simulink model "NL_Trajectory_Tracking_and_Posture_Regulation2_2024b"  (R2025b)
settings: Solver=FixedStepAuto  StartTime=0.0  StopTime=30  FixedStep=0.001  RelTol=1e-3
values from neighbouring files (symbols this model uses):
  b = 3    [NonLin_Traj_params.mat]    (also in compare_methods.m = 15; simulation.m = 500; tuning_simulation.m = 0.005)
  k1 = 0.5    [Posture_gains.mat]    (also in simulation.m = 1.5)
  k2 = 5    [Posture_gains.mat]    (also in simulation.m = 4)
  k3 = 2    [Posture_gains.mat]    (also in simulation.m = 1.5)
  last_t = size(xy, 1)-1    [simulation.m]
  theta0 = -pi/2    (= -1.57079632679)    [automated_tuning_simulation.m]    (also in regulation_tuning_simulation.m = 0.785398163397; simulation.m = 0.785398163397; tuning_simulation.m = 0.785398163397)
  x0 = S.traj.xy(1,1)    [automated_tuning_simulation.m]    (also in regulation_tuning_simulation.m = -0.8; simulation.m; tuning_simulation.m)
  x_box = 850    [parking_box.mat]    (also in regulation_tuning_simulation.m = 0; replay_q_timeseries_on_maze_pacman.m; replay_q_timeseries_on_maze_pacman_real.m; simulation.m)
  xi = 0.7    [Lin_Traj_params.mat]    (also in NonLin_Traj_params.mat = 0.706; automated_tuning_simulation.m = XI_test(j); compare_methods.m = 0.706; simulation.m)
  y0 = S.traj.xy(1,2)    [automated_tuning_simulation.m]    (also in regulation_tuning_simulation.m = 0.5; simulation.m; tuning_simulation.m)
  y_box = 880    [parking_box.mat]    (also in regulation_tuning_simulation.m = 0; replay_q_timeseries_on_maze_pacman.m; replay_q_timeseries_on_maze_pacman_real.m; simulation.m)
settings Model: Creator=david  LastModifiedBy=david
settings DataIOCC: ReturnWorkspaceOutputs=off

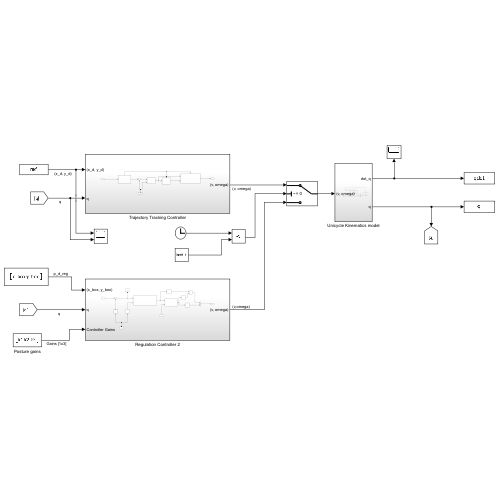
[thumbnail: Simulink's stored preview of the top-level diagram]
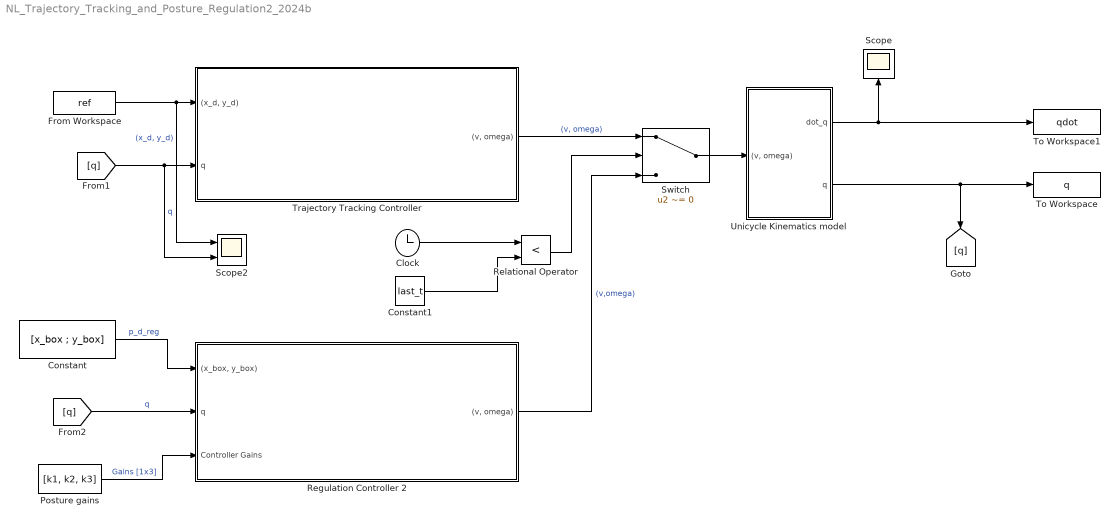
== system NL_Trajectory_Tracking_and_Posture_Regulation2_2024b ==
  Clock : Clock
  Constant : Constant  Value=[x_box ; y_box]
  Constant1 : Constant  Value=last_t
  From Workspace : FromWorkspace  VariableName=ref  OutDataTypeStr=double  SampleTime=-1
  Posture gains : Constant  Value=[k1, k2, k3]
  Regulation Controller 2 : Subsystem
  Relational Operator : RelationalOperator  Operator=<  OutDataTypeStr=boolean  RndMeth=Simplest  InputSameDT=off
  Scope : Scope
      settings: ActiveDisplayYMinimum=-1203.295  ActiveDisplayYMaximum=630.9359
  Scope2 : Scope  NumInputPorts=2
      settings: ActiveDisplayYMinimum=-704.7353  ActiveDisplayYMaximum=6091.8367  DataLoggingVariableName=ScopeData2
  Switch : Switch  Criteria=u2 ~= 0  Threshold=110  SaturateOnIntegerOverflow=off  InputSameDT=off
  To Workspace : ToWorkspace  VariableName=q  SaveFormat=Timeseries  SampleTime=-1
  To Workspace1 : ToWorkspace  VariableName=qdot  SaveFormat=Timeseries  SampleTime=-1
  Trajectory Tracking Controller : Subsystem
  Unicycle Kinematics model : Subsystem
  wires:
  Constant/1 -> Regulation Controller 2/1("(x_box, y_box)")  "p_d_reg"
  Unicycle Kinematics model/2(q) -> To Workspace/1, [q]
  From Workspace/1 -> Scope2/1, Trajectory Tracking Controller/1("(x_d, y_d)")  "(x_d, y_d)"
  Switch/1 -> Unicycle Kinematics model/1("(v, omega)")
  [q] -> Scope2/2, Trajectory Tracking Controller/2(q)  "q"
  Trajectory Tracking Controller/1("(v, omega)") -> Switch/1  "(v, omega)"
  Relational Operator/1 -> Switch/2
  Unicycle Kinematics model/1(dot_q) -> Scope/1, To Workspace1/1
  Regulation Controller 2/1("(v, omega)") -> Switch/3  "(v,omega)"
  Clock/1 -> Relational Operator/1
  Posture gains/1 -> Regulation Controller 2/3(Controller Gains)  "Gains [1x3]"
  [q] -> Regulation Controller 2/2(q)  "q"
  Constant1/1 -> Relational Operator/2

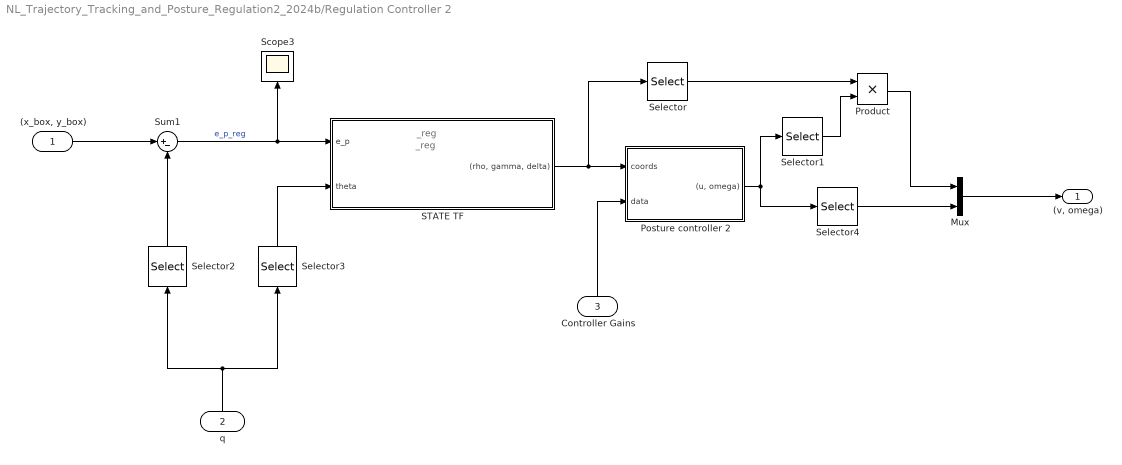
== system NL_Trajectory_Tracking_and_Posture_Regulation2_2024b/Regulation Controller 2 ==
  note: _reg
  note: _reg
  "(x_box, y_box)" : Inport
  q : Inport  Port=2
  Controller Gains : Inport  Port=3
  Mux : Mux  Inputs=2
  Posture controller 2 : Subsystem
  Product : Product
  "STATE TF " : Subsystem
  Scope3 : Scope
      settings: ActiveDisplayYMinimum=-1.51842483246E+7  ActiveDisplayYMaximum=1.6973761395E+6  DataLoggingVariableName=ScopeData3
  Selector : Selector  InputPortWidth=3  IndexOptions=Index vector (dialog)  Indices=[1]  OutputSizes=1
  Selector1 : Selector  InputPortWidth=2  IndexOptions=Index vector (dialog)  Indices=[1]  OutputSizes=1
  Selector2 : Selector  InputPortWidth=3  IndexOptions=Index vector (dialog)  Indices=[1 2]  OutputSizes=1
  Selector3 : Selector  InputPortWidth=3  IndexOptions=Index vector (dialog)  Indices=[3]  OutputSizes=1
  Selector4 : Selector  InputPortWidth=2  IndexOptions=Index vector (dialog)  Indices=[2]  OutputSizes=1
  Sum1 : Sum  Inputs=|+-
  "(v, omega)" : Outport
  wires:
  Selector2/1 -> Sum1/2
  Sum1/1 -> "STATE TF "/1(e_p), Scope3/1  "e_p_reg"
  Selector3/1 -> "STATE TF "/2(theta)
  "STATE TF "/1("(rho, gamma, delta)") -> Selector/1, Posture controller 2/1(coords)
  q/1 -> Selector3/1, Selector2/1
  Controller Gains/1 -> Posture controller 2/2(data)
  "(x_box, y_box)"/1 -> Sum1/1
  Selector/1 -> Product/1
  Selector1/1 -> Product/2
  Posture controller 2/1("(u, omega)") -> Selector4/1, Selector1/1
  Mux/1 -> "(v, omega)"/1
  Product/1 -> Mux/1
  Selector4/1 -> Mux/2

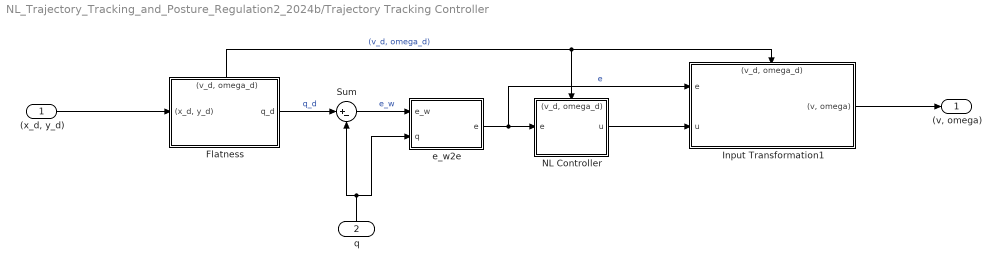
== system NL_Trajectory_Tracking_and_Posture_Regulation2_2024b/Trajectory Tracking Controller ==
  "(x_d, y_d)" : Inport
  q : Inport  Port=2
  Flatness : Subsystem
      settings: PortSchema="{\"entries\":[{\"content\":{\"sides\":[{\"content\":{\"connectorIds\":[\"In1\"]},\"type\":\"ConnectorPlacement.EquallySpacedRectSide\",\"uuid\":\"bc490c8e-5666-439b-9939-62bd84628b1f\"},{\"content\":{\"connectorIds\":[\"Out1\"],\"side\":\"RIGHT\"},\"type\":\"ConnectorPlacement.EquallySpacedRectSide\",\"uuid\":\"03a20fcc-2a82-4af2-a970-ff3426fda7d9\"},{\"content\":{\"connectorIds\":[\"Out2\"],\"side\":\"TOP\"},\"type\":\"ConnectorPlacement.EquallySpacedRectSide\",\"uuid\":\"09224fef-e39c-4959-bd2b-02867a510190\"}]},\"type\":\"ConnectorPlacement.EquallySpacedConnector\",\"uuid\":\"ad9510e9-14f7-413e-ab85-da35fb962608\"}],\"packageUris\":[\"http://schema.mathworks.com/mf0/Connector/R2020b\"],\"version\":\"1.0\"}"
  Input Transformation1 : Subsystem
      settings: PortSchema="{\"entries\":[{\"content\":{\"sides\":[{\"content\":{\"connectorIds\":[\"In1\",\"In2\"]},\"type\":\"ConnectorPlacement.EquallySpacedRectSide\",\"uuid\":\"4cbebdc1-8913-4bb0-9524-d854c819f784\"},{\"content\":{\"connectorIds\":[\"Out1\"],\"side\":\"RIGHT\"},\"type\":\"ConnectorPlacement.EquallySpacedRectSide\",\"uuid\":\"178a2b4a-0c33-47f3-8be3-bd76dfc47961\"},{\"content\":{\"connectorIds\":[\"In3\"],\"side\":\"TOP\"},\"type\":\"ConnectorPlacement.EquallySpacedRectSide\",\"uuid\":\"3e37ae07-0719-4d1d-ac53-f79374967c51\"}]},\"type\":\"ConnectorPlacement.EquallySpacedConnector\",\"uuid\":\"35111781-18f4-42cf-8750-882b65aa13c0\"}],\"packageUris\":[\"http://schema.mathworks.com/mf0/Connector/R2020b\"],\"version\":\"1.0\"}"
  NL Controller : Subsystem
      settings: PortSchema="{\"entries\":[{\"content\":{\"sides\":[{\"content\":{\"connectorIds\":[\"In1\"]},\"type\":\"ConnectorPlacement.EquallySpacedRectSide\",\"uuid\":\"111a75b0-1720-417b-bb3b-4eef3b94ce3e\"},{\"content\":{\"connectorIds\":[\"Out1\"],\"side\":\"RIGHT\"},\"type\":\"ConnectorPlacement.EquallySpacedRectSide\",\"uuid\":\"fd08faf2-16f9-4b1a-8555-2743d2eb322e\"},{\"content\":{\"connectorIds\":[\"In2\"],\"side\":\"TOP\"},\"type\":\"ConnectorPlacement.EquallySpacedRectSide\",\"uuid\":\"17cbf3ba-8c3f-4714-857c-1066f0d359bd\"}]},\"type\":\"ConnectorPlacement.EquallySpacedConnector\",\"uuid\":\"cf97b092-2f26-4cb4-9c58-7f62a3040eca\"}],\"packageUris\":[\"http://schema.mathworks.com/mf0/Connector/R2020b\"],\"version\":\"1.0\"}"
  Sum : Sum  Inputs=|+-
  e_w2e : MATLAB Function  TreatAsAtomicUnit=on
  "(v, omega)" : Outport
  wires:
  q/1 -> e_w2e/2(q), Sum/2
  NL Controller/1(u) -> Input Transformation1/2(u)
  e_w2e/1(e) -> NL Controller/1(e), Input Transformation1/1(e)  "e"
  Sum/1 -> e_w2e/1(e_w)  "e_w"
  Input Transformation1/1("(v, omega)") -> "(v, omega)"/1
  Flatness/2("(v_d, omega_d)") -> Input Transformation1/3("(v_d, omega_d)"), NL Controller/2("(v_d, omega_d)")  "(v_d, omega_d)"
  Flatness/1(q_d) -> Sum/1  "q_d"
  "(x_d, y_d)"/1 -> Flatness/1("(x_d, y_d)")

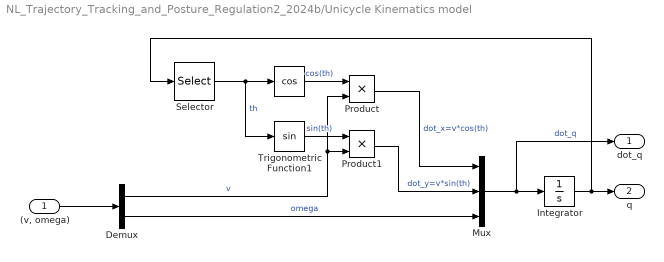
== system NL_Trajectory_Tracking_and_Posture_Regulation2_2024b/Unicycle Kinematics model ==
  "(v, omega)" : Inport
  " " : Trigonometry  Operator=cos
  Demux : Demux  Outputs=2
  Integrator : Integrator  InitialCondition=[x0; y0; theta0]
  Mux : Mux  Inputs=3
  Product : Product
  Product1 : Product
  Selector : Selector  InputPortWidth=3  IndexOptions=Index vector (dialog)  Indices=[3]  OutputSizes=1
  Trigonometric Function1 : Trigonometry
  dot_q : Outport
  q : Outport  Port=2
  wires:
  Integrator/1 -> Selector/1, q/1
  "(v, omega)"/1 -> Demux/1
  Mux/1 -> Integrator/1, dot_q/1  "dot_q"
  Demux/2 -> Mux/3  "omega"
  Selector/1 -> Trigonometric Function1/1, " "/1  "th"
  " "/1 -> Product/1  "cos(th)"
  Trigonometric Function1/1 -> Product1/1  "sin(th)"
  Demux/1 -> Product1/2, Product/2  "v"
  Product1/1 -> Mux/2  "dot_y=v*sin(th)"
  Product/1 -> Mux/1  "dot_x=v*cos(th)"

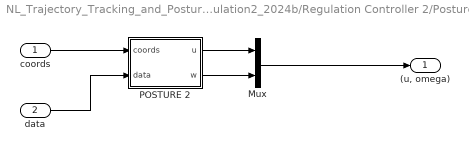
== system NL_Trajectory_Tracking_and_Posture_Regulation2_2024b/Regulation Controller 2/Posture controller 2 ==
  coords : Inport
  data : Inport  Port=2
  Mux : Mux  Inputs=2
  POSTURE 2 : MATLAB Function  TreatAsAtomicUnit=on
  "(u, omega)" : Outport
  wires:
  POSTURE 2/2(w) -> Mux/2
  coords/1 -> POSTURE 2/1(coords)
  Mux/1 -> "(u, omega)"/1
  data/1 -> POSTURE 2/2(data)
  POSTURE 2/1(u) -> Mux/1

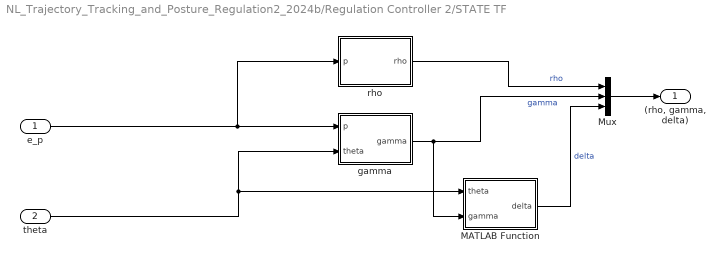
== system NL_Trajectory_Tracking_and_Posture_Regulation2_2024b/Regulation Controller 2/STATE TF  ==
  e_p : Inport
  theta : Inport  Port=2
  MATLAB Function : MATLAB Function  TreatAsAtomicUnit=on
  Mux : Mux  Inputs=3
  gamma : MATLAB Function  TreatAsAtomicUnit=on
  rho : MATLAB Function  TreatAsAtomicUnit=on
  "(rho, gamma, delta)" : Outport
  wires:
  gamma/1(gamma) -> Mux/2, MATLAB Function/2(gamma)  "gamma"
  rho/1(rho) -> Mux/1  "rho"
  MATLAB Function/1(delta) -> Mux/3  "delta"
  Mux/1 -> "(rho, gamma, delta)"/1
  e_p/1 -> rho/1(p), gamma/1(p)
  theta/1 -> MATLAB Function/1(theta), gamma/2(theta)

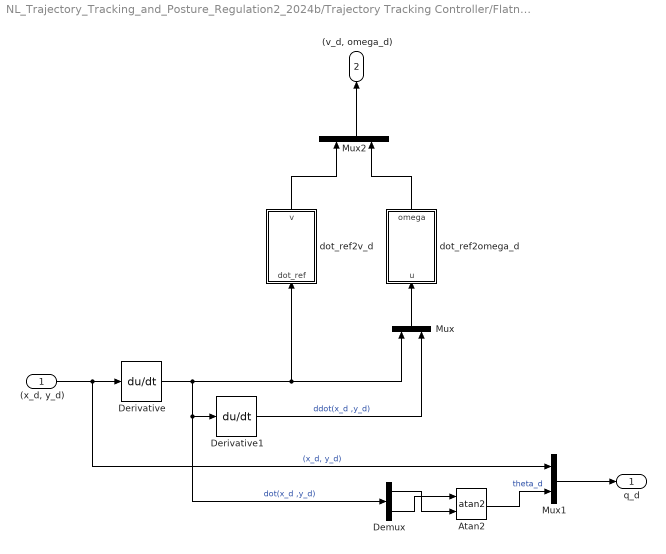
== system NL_Trajectory_Tracking_and_Posture_Regulation2_2024b/Trajectory Tracking Controller/Flatness ==
  "(x_d, y_d)" : Inport
  Atan2 : Trigonometry  Operator=atan2
  Demux : Demux  Outputs=2
  Derivative : Derivative
  Derivative1 : Derivative
  Mux : Mux  Inputs=2
  Mux1 : Mux  Inputs=2
  Mux2 : Mux  Inputs=2
  dot_ref2omega_d : MATLAB Function  TreatAsAtomicUnit=on
  dot_ref2v_d : MATLAB Function  TreatAsAtomicUnit=on
  q_d : Outport
  "(v_d, omega_d)" : Outport  Port=2
  wires:
  Atan2/1 -> Mux1/2  "theta_d"
  "(x_d, y_d)"/1 -> Mux1/1, Derivative/1  "(x_d, y_d)"
  Mux/1 -> dot_ref2omega_d/1(u)
  Derivative/1 -> Mux/1, dot_ref2v_d/1(dot_ref), Demux/1, Derivative1/1  "dot(x_d ,y_d)"
  Demux/1 -> Atan2/2
  Derivative1/1 -> Mux/2  "ddot(x_d ,y_d)"
  Demux/2 -> Atan2/1
  Mux1/1 -> q_d/1
  Mux2/1 -> "(v_d, omega_d)"/1
  dot_ref2omega_d/1(omega) -> Mux2/2
  dot_ref2v_d/1(v) -> Mux2/1

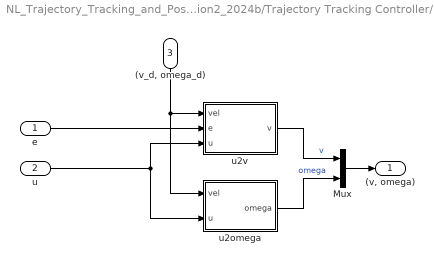
== system NL_Trajectory_Tracking_and_Posture_Regulation2_2024b/Trajectory Tracking Controller/Input Transformation1 ==
  e : Inport
  u : Inport  Port=2
  "(v_d, omega_d)" : Inport  Port=3
  Mux : Mux  Inputs=2
  u2omega : MATLAB Function  TreatAsAtomicUnit=on
  u2v : MATLAB Function  TreatAsAtomicUnit=on
  "(v, omega)" : Outport
  wires:
  e/1 -> u2v/2(e)
  Mux/1 -> "(v, omega)"/1
  u2omega/1(omega) -> Mux/2  "omega"
  u2v/1(v) -> Mux/1  "v"
  u/1 -> u2omega/2(u), u2v/3(u)
  "(v_d, omega_d)"/1 -> u2v/1(vel), u2omega/1(vel)

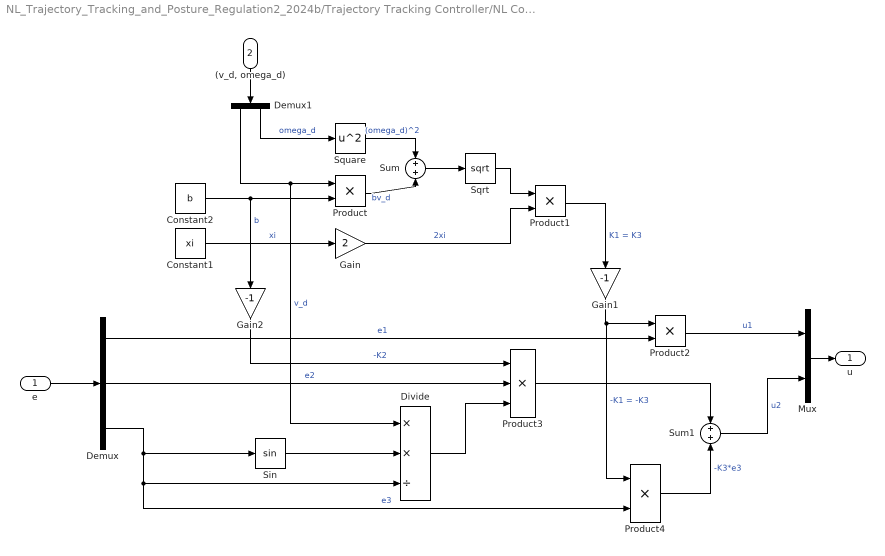
== system NL_Trajectory_Tracking_and_Posture_Regulation2_2024b/Trajectory Tracking Controller/NL Controller ==
  e : Inport
  "(v_d, omega_d)" : Inport  Port=2
  Constant1 : Constant  Value=xi
  Constant2 : Constant  Value=b
  Demux : Demux  Outputs=3
  Demux1 : Demux  Outputs=2
  Divide : Product  Inputs=**/
  Gain : Gain  Gain=2
  Gain1 : Gain  Gain=-1
  Gain2 : Gain  Gain=-1
  Mux : Mux  Inputs=2
  Product{,1..2,4} (4 alike) : Product
  Product3 : Product  Inputs=3
  Sin : Trigonometry
  Sqrt : Sqrt
  Square : Math  Operator=square
  Sum : Sum  Inputs=+|+
  Sum1 : Sum  Inputs=+|+
  u : Outport
  wires:
  e/1 -> Demux/1
  Mux/1 -> u/1
  Constant1/1 -> Gain/1  "xi"
  "(v_d, omega_d)"/1 -> Demux1/1
  Demux1/1 -> Divide/1, Product/1  "v_d"
  Constant2/1 -> Gain2/1, Product/2  "b"
  Demux1/2 -> Square/1  "omega_d"
  Square/1 -> Sum/1  "(omega_d)^2"
  Product/1 -> Sum/2  "bv_d"
  Sum/1 -> Sqrt/1
  Sqrt/1 -> Product1/1
  Gain/1 -> Product1/2  "2xi"
  Product2/1 -> Mux/1  "u1"
  Demux/1 -> Product2/2  "e1"
  Product1/1 -> Gain1/1  "K1 = K3"
  Gain1/1 -> Product2/1, Product4/1  "-K1 = -K3"
  Demux/3 -> Product4/2, Divide/3, Sin/1  "e3"
  Sin/1 -> Divide/2
  Demux/2 -> Product3/2  "e2"
  Divide/1 -> Product3/3
  Gain2/1 -> Product3/1  "-K2"
  Product3/1 -> Sum1/1
  Product4/1 -> Sum1/2  "-K3*e3"
  Sum1/1 -> Mux/2  "u2"

== matlab function NL_Trajectory_Tracking_and_Posture_Regulation2_2024b/Trajectory Tracking Controller/Flatness/dot_ref2v_d ==
  data: dot_ref input; v output
function v = fcn(dot_ref)
    dot_x = dot_ref(1);
    dot_y = dot_ref(2);

    v = sqrt(dot_x^2 + dot_y^2);

    v_min = 1e-6;
    if ~isfinite(v) || v < v_min
        v = v_min;
    end
end

== matlab function NL_Trajectory_Tracking_and_Posture_Regulation2_2024b/Trajectory Tracking Controller/e_w2e ==
  data: e_w input; e output; q input
function e = fcn(e_w, q)
    theta = q(3);

    R = [cos(theta) sin(theta) 0; 
        -sin(theta) cos(theta) 0;
             0          0      1];

    e = R*e_w;

== matlab function NL_Trajectory_Tracking_and_Posture_Regulation2_2024b/Regulation Controller 2/STATE TF /MATLAB Function ==
  data: theta input; delta output; gamma input
function delta = fcn(theta, gamma)



delta = theta + gamma;
end

== matlab function NL_Trajectory_Tracking_and_Posture_Regulation2_2024b/Trajectory Tracking Controller/Input Transformation1/u2omega ==
  data: vel input; u input; omega output
function omega = fcn(vel,u)
    omega_d = vel(2);

    omega = omega_d-u(2);

== matlab function NL_Trajectory_Tracking_and_Posture_Regulation2_2024b/Trajectory Tracking Controller/Input Transformation1/u2v ==
  data: vel input; e input; u input; v output
function v = fcn(vel, e, u)
 v_d = vel(1);

 v = v_d*cos(e(3))-u(1);

== matlab function NL_Trajectory_Tracking_and_Posture_Regulation2_2024b/Regulation Controller 2/Posture controller 2/POSTURE 2 ==
  data: u output; coords input; w output; data input
function [u,w]= fcn(coords, data)

K1 = data(1);
K2 = data(2);
K3 = data(3);

%rho = coords(1);
gamma = coords(2);
delta = coords(3);

u = K1 * cos(gamma); % u = v / rho

if abs(gamma) < 1e-6
    s = 1;                 % sin(gamma)/gamma -> 1
else
    s = sin(gamma)/gamma;
end
w = K2*gamma + K1*(s*cos(gamma))*(gamma + K3*delta);

== matlab function NL_Trajectory_Tracking_and_Posture_Regulation2_2024b/Regulation Controller 2/STATE TF /gamma ==
  data: p input; gamma output; theta input
function gamma = fcn(p, theta)

e_x = -p(1);
e_y = -p(2);

gamma = atan2(e_y,e_x) + pi - theta;

end

== matlab function NL_Trajectory_Tracking_and_Posture_Regulation2_2024b/Regulation Controller 2/STATE TF /rho ==
  data: rho output; p input
function rho = fcn(p)
e_x = -p(1);
e_y = -p(2);
rho = sqrt(e_x^2 + e_y^2);
end

== matlab function NL_Trajectory_Tracking_and_Posture_Regulation2_2024b/Trajectory Tracking Controller/Flatness/dot_ref2omega_d ==
  data: u input; omega output
function omega = fcn(u)
    dot_x  = u(1);
    dot_y  = u(2);
    ddot_x = u(3);
    ddot_y = u(4);

    den = dot_x^2 + dot_y^2;

    % Guard against singularity / non-finite inputs
    eps_den = 1e-6;
    if ~isfinite(den) || den < eps_den
        omega = 0;             % safe default at standstill
        return;
    end

    num = dot_x*ddot_y - dot_y*ddot_x;

    if ~isfinite(num)
        omega = 0;
        return;
    end

    omega = num / den;

    % clamp extreme values
    omega_max = 20;            % rad/s
    if omega > omega_max
        omega = omega_max;
    elseif omega < -omega_max
        omega = -omega_max;
    end
end
